simulink model "test_tmp"  (R2023b)
settings: Solver=FixedStepAuto  StartTime=0.0  StopTime=3  FixedStep=0.001  RelTol=1e-3
settings Model: Creator=farfar  LastModifiedBy=farfar
settings DataIOCC: ReturnWorkspaceOutputs=off

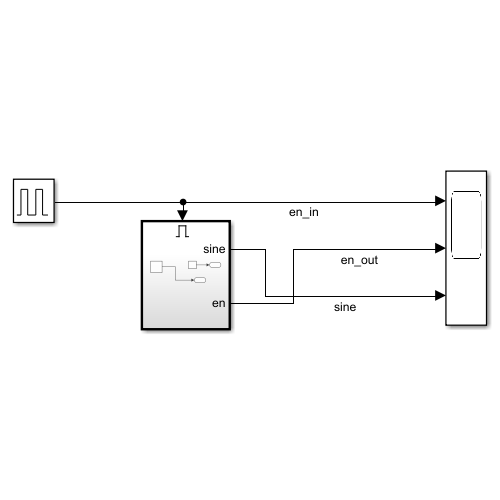
[thumbnail: Simulink's stored preview of the top-level diagram]
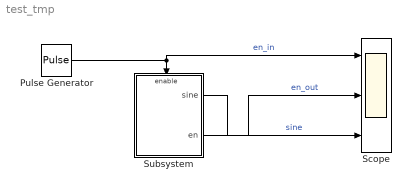
== system test_tmp ==
  Pulse Generator : DiscretePulseGenerator  PulseType=Time based  PulseWidth=50
  Scope : Scope  NumInputPorts=3
  Subsystem : Subsystem
  wires:
  Pulse Generator/1 -> Subsystem/Enable, Scope/1  "en_in"
  Subsystem/1(sine) -> Scope/3  "sine"
  Subsystem/2(en) -> Scope/2  "en_out"

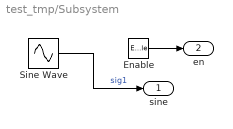
== system test_tmp/Subsystem ==
  Enable : EnablePort  StatesWhenEnabling=reset  ShowOutputPort=on
  Sine Wave : Sin  Frequency=4*2*pi  SampleTime=0.001
  sine : Outport
  en : Outport  Port=2
  wires:
  Sine Wave/1 -> sine/1  "sig1"
  Enable/1 -> en/1
